simulink model "CMV3_phase"  (R2023a)
settings: Solver=FixedStepAuto  StartTime=0.0  StopTime=1/ffund  FixedStep=1e-8  RelTol=1e-3
InitFcn:
  | fsw=50e3;
  | 
  | ma=1.15;
  | 
  | ffund=100;
  | 
  | sym= pi/6;
settings Model: Creator=enesa  LastModifiedBy=enesa

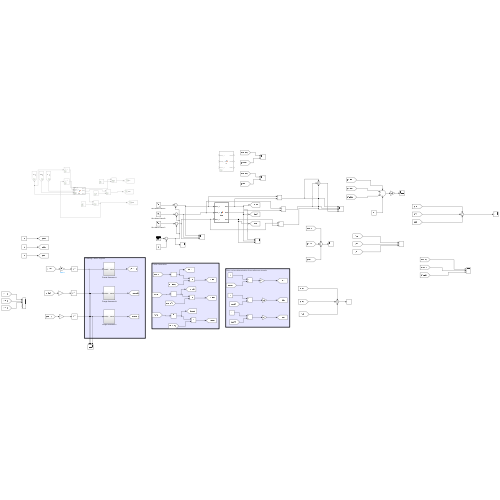
[thumbnail: Simulink's stored preview of the top-level diagram]
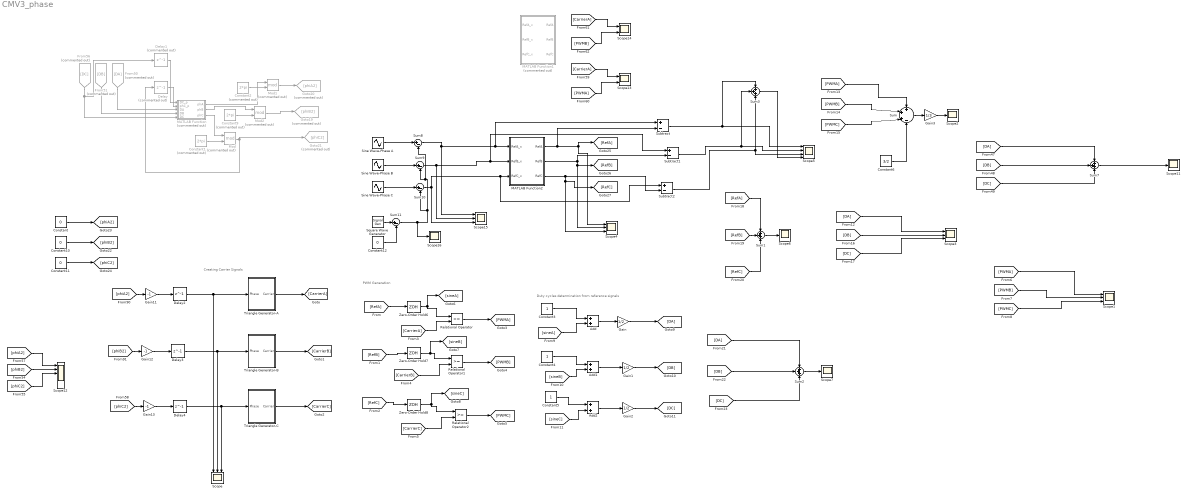
== system CMV3_phase ==
  note: Duty cycles determination from reference signals
  note: PWM Generation
  note: Creating Carrier Signals
  Add : Sum
  Add1 : Sum
  Add2 : Sum
  Constant{,10..12} (4 alike) : Constant  Value=0
  Constant1 : Constant  Commented=on  Value=2*pi
  Constant2 : Constant  Commented=on  Value=2*pi
  Constant3 : Constant
  Constant4 : Constant
  Constant5 : Constant
  Constant6 : Constant  Value=3/2
  Constant9 : Constant  Commented=on  Value=2*pi
  Delay : Delay  Commented=on  DelayLength=1  SampleTime=1/fsw
  Delay1 : Delay  Commented=on  DelayLength=1  SampleTime=1/fsw
  Delay2 : Delay  DelayLength=1  SampleTime=1/fsw
  Delay3 : Delay  DelayLength=1  SampleTime=1/fsw
  Delay4 : Delay  DelayLength=1  SampleTime=1/fsw
  From50 : From  Commented=on  GotoTag=DA
  From51 : From  Commented=on  GotoTag=DB
  From56 : From  Commented=on  GotoTag=DC
  Gain : Gain  Gain=1/2
  Gain1 : Gain  Gain=1/2
  Gain11 : Gain  Gain=-1
  Gain12 : Gain  Gain=-1
  Gain13 : Gain  Gain=-1
  Gain2 : Gain  Gain=1/2
  Gain3 : Gain  Gain=1/3
  Goto19 : Goto  Commented=on  GotoTag=phiB2
  Goto20 : Goto  Commented=on  GotoTag=phiA2
  Goto21 : Goto  Commented=on  GotoTag=phiC2
  MATLAB Function : MATLAB Function  Commented=on  TreatAsAtomicUnit=on
  MATLAB Function1 : MATLAB Function  Commented=on  TreatAsAtomicUnit=on
  MATLAB Function2 : MATLAB Function  TreatAsAtomicUnit=on
  Mod : Math  Commented=on  Operator=mod
  Mod1 : Math  Commented=on  Operator=mod
  Mod2 : Math  Commented=on  Operator=mod
  Relational Operator : RelationalOperator  OutDataTypeStr=boolean  RndMeth=Simplest  InputSameDT=off
  Relational Operator1 : RelationalOperator  OutDataTypeStr=boolean  RndMeth=Simplest  InputSameDT=off
  Relational Operator2 : RelationalOperator  OutDataTypeStr=boolean  RndMeth=Simplest  InputSameDT=off
  Scope{,1,3..4,15} (5 alike) : Scope  NumInputPorts=3
  Scope{2,6..7,11,16} (5 alike) : Scope
  Scope12 : Scope  NumInputPorts=6
  Scope13 : Scope  NumInputPorts=2
  Scope14 : Scope  NumInputPorts=2
  Scope5 : Scope  NumInputPorts=4
  Sine Wave-Phase A : Sin  Amplitude=ma  Frequency=2*pi*ffund  SampleTime=0
  Sine Wave-Phase B : Sin  Amplitude=ma  Frequency=2*pi*ffund  Phase=2*pi/3  SampleTime=0
  Sine Wave-Phase C : Sin  Amplitude=ma  Frequency=2*pi*ffund  Phase=-2*pi/3  SampleTime=0
  Square Wave Generator : SignalGenerator  WaveForm=square  Amplitude=1/3  Frequency=3*ffund
  Subtract : Sum  Inputs=+-
  Subtract1 : Sum  Inputs=+-
  Subtract2 : Sum  Inputs=+-
  Sum : Sum  Inputs=+++-
  Sum{1..3,7} (4 alike) : Sum  Inputs=+++
  Sum{8..11} (4 alike) : Sum  Inputs=|+-
  Triangle Generator-A : Subsystem
  Triangle Generator-B : Subsystem
  Triangle Generator-C : Subsystem
  Zero-Order Hold6 : ZeroOrderHold  SampleTime=5/fsw
  Zero-Order Hold7 : ZeroOrderHold  SampleTime=5/fsw
  Zero-Order Hold8 : ZeroOrderHold  SampleTime=5/fsw
  wires:
  [PWMA] -> Scope1/1
  [PWMB] -> Scope1/2
  [PWMC] -> Scope1/3
  [PWMA] -> Sum/1
  [PWMB] -> Sum/2
  [PWMC] -> Sum/3
  Sum/1 -> Gain3/1
  Gain3/1 -> Scope2/1
  Constant6/1 -> Sum/4
  [DA] -> Scope3/1
  [DB] -> Scope3/2
  [DC] -> Scope3/3
  Triangle Generator-C/1(Carrier) -> [CarrierC]
  Triangle Generator-B/1(Carrier) -> [CarrierB]
  Triangle Generator-A/1(Carrier) -> [CarrierA]
  [CarrierB] -> Relational Operator1/2
  Relational Operator1/1 -> [PWMB]
  Relational Operator/1 -> [PWMA]
  Relational Operator2/1 -> [PWMC]
  [CarrierC] -> Relational Operator2/2
  [RefA] -> Zero-Order Hold6/1
  [RefC] -> Zero-Order Hold8/1
  [CarrierA] -> Relational Operator/2
  [RefB] -> Zero-Order Hold7/1
  [sineC] -> Add2/2
  Constant4/1 -> Add1/1
  Constant3/1 -> Add/1
  Add2/1 -> Gain2/1
  Gain/1 -> [DA]
  Gain2/1 -> [DC]
  Add1/1 -> Gain1/1
  [sineB] -> Add1/2
  Constant5/1 -> Add2/1
  [sineA] -> Add/2
  Gain1/1 -> [DB]
  Add/1 -> Gain/1
  [DA] -> Sum7/1
  [DC] -> Sum7/3
  [DB] -> Sum7/2
  Sum7/1 -> Scope11/1
  [phiB2] -> Scope12/2
  [phiC2] -> Scope12/3
  From50/1 -> MATLAB Function/3(DA)
  From51/1 -> MATLAB Function/4(DB)
  From56/1 -> Delay1/1, MATLAB Function/5(DC)
  [phiA2] -> Scope12/1
  [CarrierA] -> Scope13/1
  [PWMA] -> Scope13/2
  [CarrierA] -> Scope14/1
  [PWMB] -> Scope14/2
  Constant1/1 -> Mod/2
  Constant2/1 -> Mod1/2
  Constant9/1 -> Mod2/2
  Mod2/1 -> Goto19/1
  Mod/1 -> Delay/1, Goto21/1
  Mod1/1 -> Goto20/1
  MATLAB Function/1(phA) -> Mod1/1
  MATLAB Function/2(phB) -> Mod2/1
  MATLAB Function/3(phC) -> Mod/1
  [phiA2] -> Gain11/1
  [phiB2] -> Gain12/1
  [phiC2] -> Gain13/1
  Gain11/1 -> Delay2/1
  Gain13/1 -> Delay4/1
  Zero-Order Hold6/1 -> Relational Operator/1, [sineA]
  Zero-Order Hold7/1 -> [sineB], Relational Operator1/1
  Zero-Order Hold8/1 -> Relational Operator2/1, [sineC]
  Gain12/1 -> Delay3/1
  Delay/1 -> MATLAB Function/2(phC_p)
  Delay1/1 -> MATLAB Function/1(DC_p)
  Delay2/1 -> Triangle Generator-A/1(Phase), Scope/1
  Delay3/1 -> Triangle Generator-B/1(Phase), Scope/2
  Delay4/1 -> Triangle Generator-C/1(Phase), Scope/3
  Constant/1 -> [phiA2]
  Constant11/1 -> [phiC2]
  Constant10/1 -> [phiB2]
  Sine Wave-Phase A/1 -> Sum8/1
  Sum8/1 -> MATLAB Function2/1(RefA_x), Subtract/1, Scope15/1
  Sine Wave-Phase B/1 -> Sum9/1
  Sine Wave-Phase C/1 -> Sum10/1
  Sum10/1 -> Scope15/3, MATLAB Function2/3(RefC_x), Subtract2/1
  Square Wave Generator/1 -> Sum11/1
  Sum11/1 -> Scope16/1, Sum10/2, Sum8/2, Sum9/2
  Constant12/1 -> Sum11/2
  MATLAB Function2/2(RefB) -> Scope4/2, [RefB], Subtract1/2
  MATLAB Function2/1(RefA) -> Subtract/2, [RefA], Scope4/1
  MATLAB Function2/3(RefC) -> Subtract2/2, Scope4/3, [RefC]
  Sum9/1 -> MATLAB Function2/2(RefB_x), Subtract1/1, Scope15/2
  Subtract/1 -> Sum3/1, Scope5/1
  Subtract1/1 -> Sum3/2, Scope5/2
  Subtract2/1 -> Sum3/3, Scope5/3
  [RefA] -> Sum1/1
  [RefB] -> Sum1/2
  [RefC] -> Sum1/3
  Sum1/1 -> Scope6/1
  [DA] -> Sum2/1
  [DB] -> Sum2/2
  [DC] -> Sum2/3
  Sum2/1 -> Scope7/1
  Sum3/1 -> Scope5/4

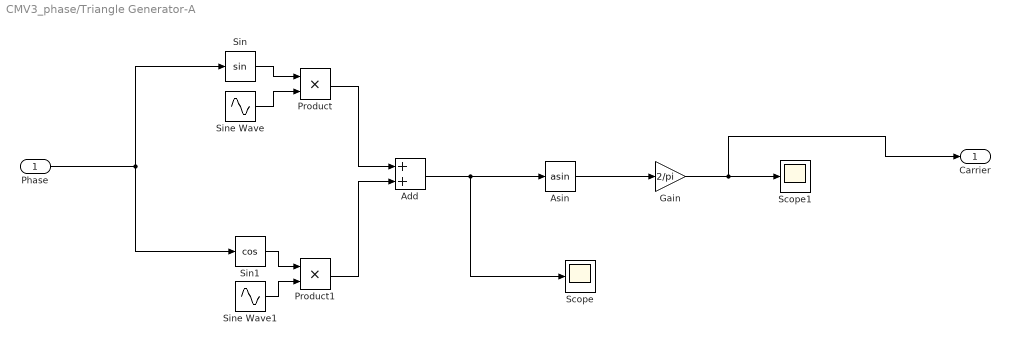
== system CMV3_phase/Triangle Generator-A ==
  Phase : Inport
  Add : Sum
  Asin : Trigonometry  Operator=asin
  Gain : Gain  Gain=2/pi
  Product : Product
  Product1 : Product
  Scope : Scope
  Scope1 : Scope
  Sin : Trigonometry
  Sin1 : Trigonometry  Operator=cos
  Sine Wave : Sin  Frequency=2*pi*fsw  SampleTime=0
  Sine Wave1 : Sin  Frequency=2*pi*fsw  Phase=-pi/2  SampleTime=0
  Carrier : Outport
  wires:
  Sin/1 -> Product/1
  Sine Wave/1 -> Product/2
  Phase/1 -> Sin/1, Sin1/1
  Product/1 -> Add/1
  Asin/1 -> Gain/1
  Gain/1 -> Carrier/1, Scope1/1
  Sine Wave1/1 -> Product1/2
  Product1/1 -> Add/2
  Add/1 -> Asin/1, Scope/1
  Sin1/1 -> Product1/1

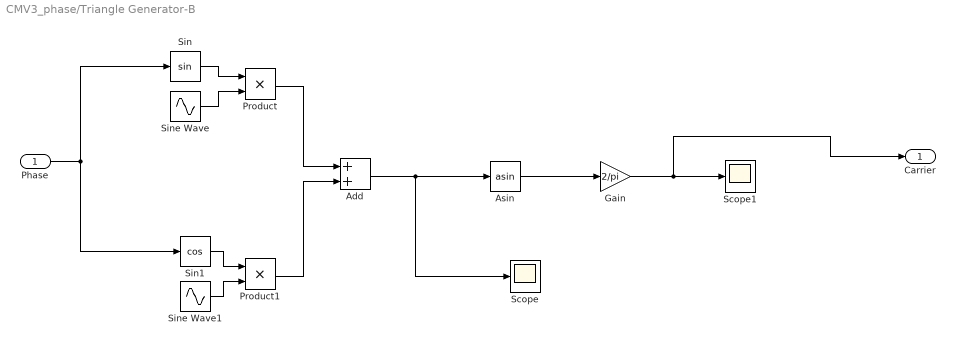
== system CMV3_phase/Triangle Generator-B ==
  Phase : Inport
  Add : Sum
  Asin : Trigonometry  Operator=asin
  Gain : Gain  Gain=2/pi
  Product : Product
  Product1 : Product
  Scope : Scope
  Scope1 : Scope
  Sin : Trigonometry
  Sin1 : Trigonometry  Operator=cos
  Sine Wave : Sin  Frequency=2*pi*fsw  SampleTime=0
  Sine Wave1 : Sin  Frequency=2*pi*fsw  Phase=-pi/2  SampleTime=0
  Carrier : Outport
  wires:
  Sin/1 -> Product/1
  Sine Wave/1 -> Product/2
  Phase/1 -> Sin1/1, Sin/1
  Product/1 -> Add/1
  Asin/1 -> Gain/1
  Gain/1 -> Carrier/1, Scope1/1
  Sine Wave1/1 -> Product1/2
  Product1/1 -> Add/2
  Add/1 -> Asin/1, Scope/1
  Sin1/1 -> Product1/1

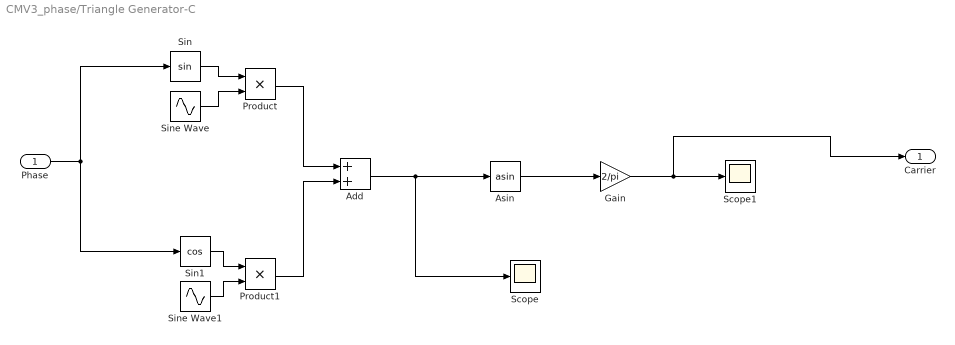
== system CMV3_phase/Triangle Generator-C ==
  Phase : Inport
  Add : Sum
  Asin : Trigonometry  Operator=asin
  Gain : Gain  Gain=2/pi
  Product : Product
  Product1 : Product
  Scope : Scope
  Scope1 : Scope
  Sin : Trigonometry
  Sin1 : Trigonometry  Operator=cos
  Sine Wave : Sin  Frequency=2*pi*fsw  SampleTime=0
  Sine Wave1 : Sin  Frequency=2*pi*fsw  Phase=-pi/2  SampleTime=0
  Carrier : Outport
  wires:
  Sin/1 -> Product/1
  Sine Wave/1 -> Product/2
  Phase/1 -> Sin1/1, Sin/1
  Product/1 -> Add/1
  Asin/1 -> Gain/1
  Gain/1 -> Carrier/1, Scope1/1
  Sine Wave1/1 -> Product1/2
  Product1/1 -> Add/2
  Add/1 -> Asin/1, Scope/1
  Sin1/1 -> Product1/1

== matlab function CMV3_phase/MATLAB Function1 ==
  data: RefA output; RefA_x input; RefB_x input; RefB output; RefC_x input; RefC output
function [RefA, RefB, RefC] = fcn(RefA_x, RefB_x, RefC_x)

RefA = RefA_x;
RefB = RefB_x;
RefC = RefC_x;

if RefA_x > 1
        RefB = RefB_x + (RefA_x - 1)/2;
        RefC = RefC_x + (RefA_x - 1)/2;
        RefA = 1; % Set RefA to 1 when RefA_x > 1
end


if RefA_x < -1
  
        RefB = RefB_x + (RefA_x +1)/2;
        RefC = RefC_x +  (RefA_x +1)/2;
        RefA = -1; % Set RefA to 1 when RefA_x > 1
end


if RefB_x > 1
   
        RefA = RefA_x + (RefB_x - 1)/2;

        RefC = RefC_x + (RefB_x - 1)/2;

    RefB = 1; % Set RefA to 1 when RefA_x > 1
end


if RefB_x < -1
   
        RefA = RefA_x + (RefB_x +1)/2;

        RefC = RefC_x + (RefB_x + 1)/2;

    RefB = -1; % Set RefA to 1 when RefA_x > 1
end

if RefC_x > 1
   
        RefA = RefA_x + (RefC_x - 1)/2;

        RefB = RefB_x + (RefC_x - 1)/2;

    RefC = 1; % Set RefA to 1 when RefA_x > 1
end


if RefC_x < -1
    
        RefA = RefA_x + (RefC_x +1)/2;

        RefB = RefB_x + (RefC_x + 1/2);

    RefC = -1; % Set RefA to 1 when RefA_x > 1
end

end

== matlab function CMV3_phase/MATLAB Function ==
  data: DC_p input; phC_p input; DA input; phA output; DB input; DC input; phB output; phC output
function [phA, phB,phC] = fcn(DC_p, phC_p, DA,DB,DC)

phA=phC_p+((DA+DC_p))*pi;
phB=phA+((DA+DB))*pi;
phC= phB+((DB+DC))*pi;

end

== matlab function CMV3_phase/MATLAB Function2 ==
  data: RefA output; RefA_x input; RefB_x input; RefB output; RefC_x input; RefC output
function [RefA, RefB, RefC] = fcn(RefA_x, RefB_x, RefC_x)

RefA = RefA_x;
RefB = RefB_x;
RefC = RefC_x;

if RefA_x > 1
    if RefB_x < 0 && RefC_x < 0
        % Both RefB_x and RefC_x are less than 0
        % Determine which one takes precedence or any other logic needed
        % For example, set RefB and RefC to 0
        RefB = 0;
        RefC = 0;
    elseif RefB_x < 0
        RefB = RefB_x + RefA_x - 1;
    elseif RefC_x < 0
        RefC = RefC_x + RefA_x - 1;
    end
    RefA = 1; % Set RefA to 1 when RefA_x > 1
end


if RefA_x < -1
    if RefB_x > 0 && RefC_x > 0
        % Both RefB_x and RefC_x are less than 0
        % Determine which one takes precedence or any other logic needed
        % For example, set RefB and RefC to 0
        RefB = 0;
        RefC = 0;
    elseif RefB_x > 0
        RefB = RefB_x + RefA_x +1;
    elseif RefC_x > 0
        RefC = RefC_x + RefA_x + 1;
    end
    RefA = -1; % Set RefA to 1 when RefA_x > 1
end


if RefB_x > 1
    if RefA_x < 0 && RefC_x < 0
        % Both RefB_x and RefC_x are less than 0
        % Determine which one takes precedence or any other logic needed
        % For example, set RefB and RefC to 0
        RefA = 0;
        RefC = 0;
    elseif RefA_x < 0
        RefA = RefA_x + RefB_x - 1;
    elseif RefC_x < 0
        RefC = RefC_x + RefB_x - 1;
    end
    RefB = 1; % Set RefA to 1 when RefA_x > 1
end


if RefB_x < -1
    if RefA_x > 0 && RefC_x > 0
        % Both RefB_x and RefC_x are less than 0
        % Determine which one takes precedence or any other logic needed
        % For example, set RefB and RefC to 0
        RefA = 0;
        RefC = 0;
    elseif RefA_x > 0
        RefA = RefA_x + RefB_x +1;
    elseif RefC_x > 0
        RefC = RefC_x + RefB_x + 1;
    end
    RefB = -1; % Set RefA to 1 when RefA_x > 1
end

if RefC_x > 1
    if RefA_x < 0 && RefB_x < 0
        % Both RefB_x and RefC_x are less than 0
        % Determine which one takes precedence or any other logic needed
        % For example, set RefB and RefC to 0
        RefA = 0;
        RefB = 0;
    elseif RefA_x < 0
        RefA = RefA_x + RefC_x - 1;
    elseif RefB_x < 0
        RefB = RefB_x + RefC_x - 1;
    end
    RefC = 1; % Set RefA to 1 when RefA_x > 1
end


if RefC_x < -1
    if RefA_x > 0 && RefB_x > 0
        % Both RefB_x and RefC_x are less than 0
        % Determine which one takes precedence or any other logic needed
        % For example, set RefB and RefC to 0
        RefA = 0;
        RefB = 0;
    elseif RefA_x > 0
        RefA = RefA_x + RefC_x +1;
    elseif RefB_x > 0
        RefB = RefB_x + RefC_x + 1;
    end
    RefC = -1; % Set RefA to 1 when RefA_x > 1
end

end
